simulink model "SVPWM"  (R2019a)
settings: Solver=VariableStepAuto  StartTime=0.0  StopTime=1.0  RelTol=1e-3
libraries: simulink x16, powerlib_meascontrol x1, powerlib x1
settings Model: Creator=Amanna  LastModifiedBy=Amanna

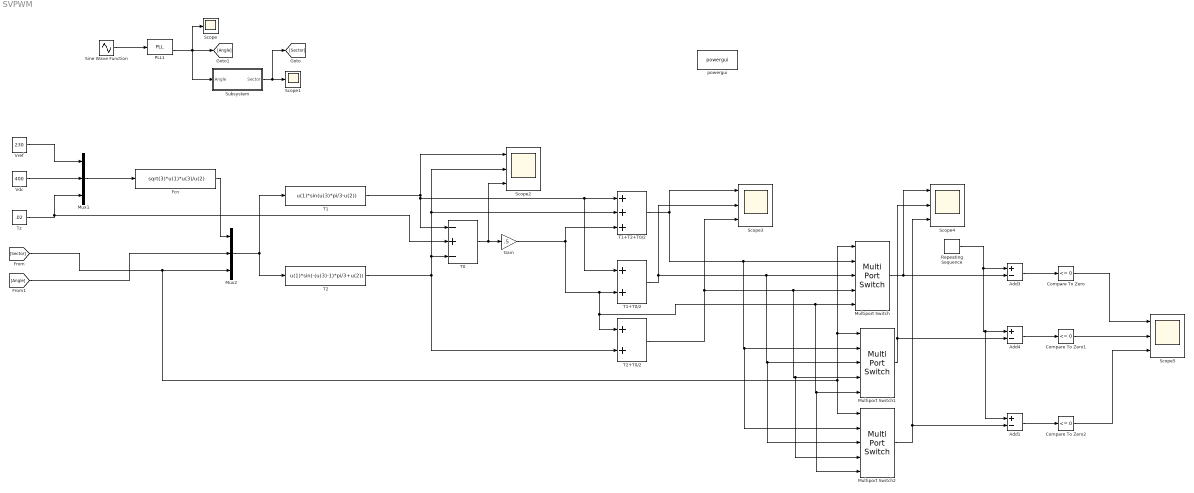
== system SVPWM ==
  Add1 : Sum  Inputs=+-
  Add3 : Sum  Inputs=+-
  Add4 : Sum  Inputs=+-
  Compare To Zero : simulink/Logic and Bit Operations/Compare To Zero  relop=<=  OutDataTypeStr=boolean
  Compare To Zero1 : simulink/Logic and Bit Operations/Compare To Zero  relop=<=  OutDataTypeStr=boolean
  Compare To Zero2 : simulink/Logic and Bit Operations/Compare To Zero  relop=<=  OutDataTypeStr=boolean
  Fcn : Fcn  Expr=sqrt(3)*u(1)*u(3)/u(2)
  Gain : Gain  Gain=.5
  Multiport Switch : MultiPortSwitch  DataPortOrder=Specify indices  Inputs=4  DataPortIndices={[1,6],2,5,[3,4]}
  Multiport Switch1 : MultiPortSwitch  DataPortOrder=Specify indices  Inputs=4  DataPortIndices={[2,3],4,1,[5,6]}
  Multiport Switch2 : MultiPortSwitch  DataPortOrder=Specify indices  Inputs=4  DataPortIndices={[4,5],6,3,[1,2]}
  Mux1 : Mux  Inputs=3
  Mux2 : Mux  Inputs=3
  "PLL1 " : powerlib_meascontrol/PLL/PLL  Fmin=45  Par_Init=[0, 60]  ParK=[180, 3200, 1]  TcD=1e-4  MaxRateChangeFreq=12  FilterCutOffFreq=25  Ts=0  AGC=on
      settings: SourceProductName=Simscape Electrical  SourceProductBaseCode=PS
  Repeating Sequence : simulink/Sources/Repeating Sequence  rep_seq_t=[0 0.001]  rep_seq_y=[0 0.02]
  Scope : Scope
  Scope1 : Scope
  Scope{2..5} (4 alike) : Scope  NumInputPorts=3
  Sine Wave Function : Sin  Frequency=2*pi*50  SampleTime=0
  Subsystem : Subsystem
  T0 : Sum  Inputs=-+-
  T1 : Fcn  Expr=u(1)*sin(u(3)*pi/3-u(2))
  T1+T0/2 : Sum  Inputs=2
  T1+T2+T0/2 : Sum  Inputs=3
  T2 : Fcn  Expr=u(1)*sin(-(u(3)-1)*pi/3+u(2))
  T2+T0/2 : Sum  Inputs=2
  Tz : Constant  Value=.02
  Vdc : Constant  Value=400
  Vref : Constant  Value=230
  powergui : powerlib/powergui  Priority=1  SimulationMode=Continuous  SampleTime=50e-6  frequency=60  Iterations=50  frequencyindice=60  Pbase=100e6  ErrMax=1e-4  UnitsV=kV  UnitsW=MW  buscounter=0  FunctionMessages=off  echomessages=off  EnableUseOfTLC=off  CurrentSourceSwitches=off  DisableSnubberDevices=off  DisableRonSwitches=on  DisableVfSwitches=off  DisplayEquations=off  AutomaticDiscreteSolvers=off  SolverType=Tustin/Backward Euler (TBE)  Interpol=off  ExternalGateDelay=off  methode=off  Ts=100  x0status=blocks  SPID=on  SwTol=0  HookPort=off  NonlinearTolerance=0  nMaxIteration=15  ContinueOnMaxIteration=off  RestoreLinks=warning  ResistiveCurrentMeasurement=off  Frange=[0:2:500]  Ylog=off  Xlog=on  ShowGrid=off  save=off  variable=ZData  structure=0  ZoomFFT=off  StartTime=0.0  cycles=1  DisplayStyle=1  fundamental=60  FreqAxis=off  MaxFrequency=1000  frequencyindicesteady=1  RmsSteady=1  display=off
      settings: SourceProductName=Simscape Electrical
  wires:
  Vref/1 -> Mux1/1
  Vdc/1 -> Mux1/2
  Mux1/1 -> Fcn/1
  "PLL1 "/2 -> [Angle], Scope/1, Subsystem/1(Angle)
  Sine Wave Function/1 -> "PLL1 "/1
  Subsystem/1(Sector) -> [Sector], Scope1/1
  Fcn/1 -> Mux2/1
  Mux2/1 -> T1/1, T2/1
  T1/1 -> T1+T0/2/1, T1+T2+T0/2/1, T0/1, Scope2/1
  T2/1 -> Scope2/2, T1+T2+T0/2/2, T0/3, T2+T0/2/2
  Tz/1 -> T0/2, Mux1/3
  T0/1 -> Scope2/3, Gain/1
  [Angle] -> Mux2/2
  [Sector] -> Multiport Switch2/1, Multiport Switch1/1, Multiport Switch/1, Mux2/3
  Gain/1 -> Multiport Switch2/5, Multiport Switch1/5, Multiport Switch/5, T2+T0/2/1, T1+T0/2/2, T1+T2+T0/2/3
  T1+T2+T0/2/1 -> Multiport Switch2/2, Multiport Switch1/2, Multiport Switch/2, Scope3/1
  T1+T0/2/1 -> Scope3/2, Multiport Switch2/3, Multiport Switch1/3, Multiport Switch/3
  T2+T0/2/1 -> Scope3/3, Multiport Switch2/4, Multiport Switch1/4, Multiport Switch/4
  Multiport Switch/1 -> Add3/2, Scope4/1
  Multiport Switch1/1 -> Add4/2, Scope4/2
  Multiport Switch2/1 -> Scope4/3, Add1/2
  Repeating Sequence/1 -> Add3/1, Add1/1, Add4/1
  Add3/1 -> Compare To Zero/1
  Add4/1 -> Compare To Zero1/1
  Add1/1 -> Compare To Zero2/1
  Compare To Zero/1 -> Scope5/1
  Compare To Zero1/1 -> Scope5/2
  Compare To Zero2/1 -> Scope5/3

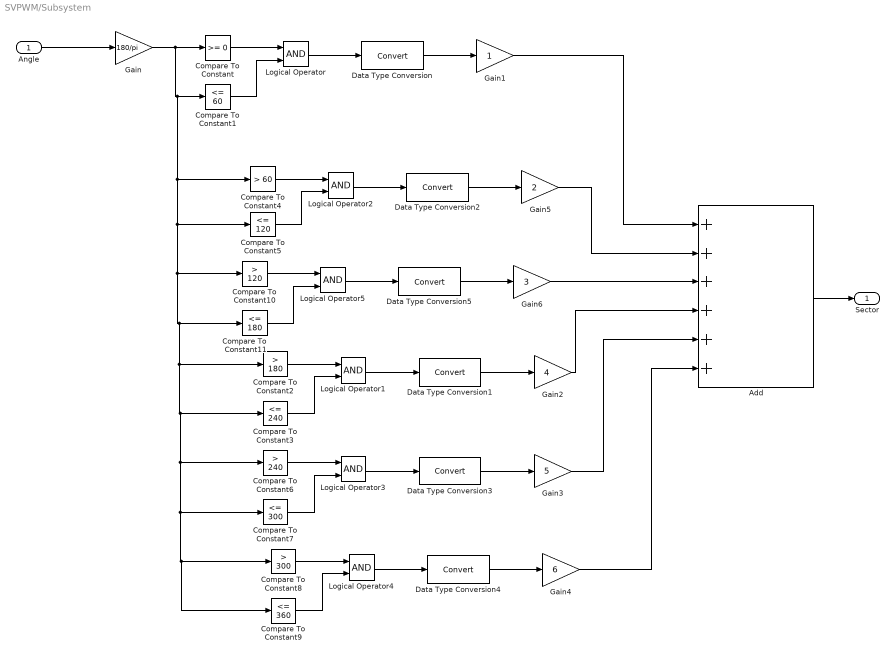
== system SVPWM/Subsystem ==
  Angle : Inport
  Add : Sum  Inputs=++++++
  Compare To Constant : simulink/Logic and Bit Operations/Compare To Constant  relop=>=  const=0  OutDataTypeStr=boolean
  Compare To Constant1 : simulink/Logic and Bit Operations/Compare To Constant  relop=<=  const=60  OutDataTypeStr=boolean
  Compare To Constant10 : simulink/Logic and Bit Operations/Compare To Constant  relop=>  const=120  OutDataTypeStr=boolean
  Compare To Constant11 : simulink/Logic and Bit Operations/Compare To Constant  relop=<=  const=180  OutDataTypeStr=boolean
  Compare To Constant2 : simulink/Logic and Bit Operations/Compare To Constant  relop=>  const=180  OutDataTypeStr=boolean
  Compare To Constant3 : simulink/Logic and Bit Operations/Compare To Constant  relop=<=  const=240  OutDataTypeStr=boolean
  Compare To Constant4 : simulink/Logic and Bit Operations/Compare To Constant  relop=>  const=60  OutDataTypeStr=boolean
  Compare To Constant5 : simulink/Logic and Bit Operations/Compare To Constant  relop=<=  const=120  OutDataTypeStr=boolean
  Compare To Constant6 : simulink/Logic and Bit Operations/Compare To Constant  relop=>  const=240  OutDataTypeStr=boolean
  Compare To Constant7 : simulink/Logic and Bit Operations/Compare To Constant  relop=<=  const=300  OutDataTypeStr=boolean
  Compare To Constant8 : simulink/Logic and Bit Operations/Compare To Constant  relop=>  const=300  OutDataTypeStr=boolean
  Compare To Constant9 : simulink/Logic and Bit Operations/Compare To Constant  relop=<=  const=360  OutDataTypeStr=boolean
  Data Type Conversion{,1..5} (6 alike) : DataTypeConversion
  Gain : Gain  Gain=180/pi
  Gain1 : Gain
  Gain2 : Gain  Gain=4
  Gain3 : Gain  Gain=5
  Gain4 : Gain  Gain=6
  Gain5 : Gain  Gain=2
  Gain6 : Gain  Gain=3
  Logical Operator{,1..5} (6 alike) : Logic  AllPortsSameDT=off  OutDataTypeStr=boolean
  Sector : Outport
  wires:
  Angle/1 -> Gain/1
  Compare To Constant/1 -> Logical Operator/1
  Compare To Constant1/1 -> Logical Operator/2
  Logical Operator/1 -> Data Type Conversion/1
  Data Type Conversion/1 -> Gain1/1
  Data Type Conversion2/1 -> Gain5/1
  Logical Operator2/1 -> Data Type Conversion2/1
  Compare To Constant4/1 -> Logical Operator2/1
  Compare To Constant5/1 -> Logical Operator2/2
  Compare To Constant3/1 -> Logical Operator1/2
  Compare To Constant2/1 -> Logical Operator1/1
  Gain/1 -> Compare To Constant4/1, Compare To Constant10/1, Compare To Constant2/1, Compare To Constant9/1, Compare To Constant8/1, Compare To Constant7/1, Compare To Constant6/1, Compare To Constant3/1, Compare To Constant11/1, Compare To Constant5/1, Compare To Constant1/1, Compare To Constant/1
  Logical Operator1/1 -> Data Type Conversion1/1
  Data Type Conversion1/1 -> Gain2/1
  Data Type Conversion5/1 -> Gain6/1
  Logical Operator5/1 -> Data Type Conversion5/1
  Compare To Constant10/1 -> Logical Operator5/1
  Compare To Constant11/1 -> Logical Operator5/2
  Compare To Constant7/1 -> Logical Operator3/2
  Compare To Constant6/1 -> Logical Operator3/1
  Logical Operator3/1 -> Data Type Conversion3/1
  Data Type Conversion3/1 -> Gain3/1
  Compare To Constant9/1 -> Logical Operator4/2
  Compare To Constant8/1 -> Logical Operator4/1
  Logical Operator4/1 -> Data Type Conversion4/1
  Data Type Conversion4/1 -> Gain4/1
  Gain1/1 -> Add/1
  Gain5/1 -> Add/2
  Gain6/1 -> Add/3
  Gain2/1 -> Add/4
  Gain3/1 -> Add/5
  Gain4/1 -> Add/6
  Add/1 -> Sector/1
